simulink model "gm_DUALportRAMinterface_v3"  (R2024a)
settings: Solver=FixedStepDiscrete  StartTime=0.0  StopTime=20  RelTol=1e-3
undefined symbols (not defined in the file or in its folder): magnitude, Ts
libraries: hdlsllib x226, hdlmdlgenlib x102, embmathops x6, simulink x1, dsphdlxfrm2 x1
(part 5 of 6)

== system gm_DUALportRAMinterface_v3/PL/integration_block1/accumulator_scorer/64bitmsb_finder/8bit_PE10 ==
  D7 : Inport  OutDataTypeStr=boolean  PortDimensions=1  SampleTime=3.00000003e-08
  D6 : Inport  Port=2  OutDataTypeStr=boolean  PortDimensions=1  SampleTime=3.00000003e-08
  D5 : Inport  Port=3  OutDataTypeStr=boolean  PortDimensions=1  SampleTime=3.00000003e-08
  D4 : Inport  Port=4  OutDataTypeStr=boolean  PortDimensions=1  SampleTime=3.00000003e-08
  D3 : Inport  Port=5  OutDataTypeStr=boolean  PortDimensions=1  SampleTime=3.00000003e-08
  D2 : Inport  Port=6  OutDataTypeStr=boolean  PortDimensions=1  SampleTime=3.00000003e-08
  D1 : Inport  Port=7  OutDataTypeStr=boolean  PortDimensions=1  SampleTime=3.00000003e-08
  D0 : Inport  Port=8  OutDataTypeStr=boolean  PortDimensions=1  SampleTime=3.00000003e-08
  Add : Sum  OutDataTypeStr=fixdt(0, 5, 0)
  Bit Concat : hdlsllib/Logic and Bit Operations/Bit Concat  numInputs=3
  Constant2 : Constant  OutDataTypeStr=fixdt(0,4,0)  SampleTime=Ts
  Constant3 : Constant  Value=0  OutDataTypeStr=fixdt(0,4,0)  SampleTime=Ts
  Logical Operator{,10..16,22} (9 alike) : Logic  Operator=NOT  IconShape=distinctive  AllPortsSameDT=off  OutDataTypeStr=boolean
  Logical Operator1 : Logic  Operator=NAND  IconShape=distinctive  AllPortsSameDT=off  OutDataTypeStr=boolean
  Logical Operator{17..20} (4 alike) : Logic  Operator=OR  Inputs=4  IconShape=distinctive  AllPortsSameDT=off  OutDataTypeStr=boolean
  Logical Operator2 : Logic  Operator=NAND  Inputs=4  IconShape=distinctive  AllPortsSameDT=off  OutDataTypeStr=boolean
  Logical Operator21 : Logic  Operator=NAND  Inputs=3  IconShape=distinctive  AllPortsSameDT=off  OutDataTypeStr=boolean
  Logical Operator23 : Logic  IconShape=distinctive  AllPortsSameDT=off  OutDataTypeStr=boolean
  Logical Operator3 : Logic  Operator=NAND  Inputs=3  IconShape=distinctive  AllPortsSameDT=off  OutDataTypeStr=boolean
  Logical Operator4 : Logic  Inputs=3  IconShape=distinctive  AllPortsSameDT=off  OutDataTypeStr=boolean
  Logical Operator5 : Logic  Inputs=3  IconShape=distinctive  AllPortsSameDT=off  OutDataTypeStr=boolean
  Logical Operator6 : Logic  Inputs=4  IconShape=distinctive  AllPortsSameDT=off  OutDataTypeStr=boolean
  Logical Operator7 : Logic  Operator=NAND  Inputs=3  IconShape=distinctive  AllPortsSameDT=off  OutDataTypeStr=boolean
  Logical Operator8 : Logic  Operator=NAND  Inputs=4  IconShape=distinctive  AllPortsSameDT=off  OutDataTypeStr=boolean
  Logical Operator9 : Logic  Operator=NAND  Inputs=4  IconShape=distinctive  AllPortsSameDT=off  OutDataTypeStr=boolean
  Switch : Switch  Criteria=u2 > Threshold  OutDataTypeStr=fixdt(0, 4, 0)  SaturateOnIntegerOverflow=off  InputSameDT=off
  data2 : Outport  SampleTime=3.00000003e-08
  valid : Outport  Port=2  SampleTime=3.00000003e-08
  wires:
  D7/1 -> Logical Operator/1
  D6/1 -> Logical Operator1/2
  D5/1 -> Logical Operator3/3
  D4/1 -> Logical Operator2/4
  D3/1 -> Logical Operator7/3
  D2/1 -> Logical Operator8/4
  D1/1 -> Logical Operator9/4
  D0/1 -> Logical Operator20/2
  Add/1 -> data2/1
  Bit Concat/1 -> Add/2
  Constant2/1 -> Switch/3
  Constant3/1 -> Switch/1
  Logical Operator/1 -> Logical Operator6/3, Logical Operator5/3, Logical Operator4/3, Logical Operator3/2, Logical Operator2/3, Logical Operator10/1, Logical Operator1/1
  Logical Operator1/1 -> Logical Operator6/2, Logical Operator5/2, Logical Operator4/2, Logical Operator3/1, Logical Operator2/2, Logical Operator11/1
  Logical Operator10/1 -> Logical Operator19/1, Logical Operator18/1, Logical Operator17/1
  Logical Operator11/1 -> Logical Operator18/2, Logical Operator17/2
  Logical Operator12/1 -> Logical Operator19/2, Logical Operator17/3
  Logical Operator13/1 -> Logical Operator17/4
  Logical Operator14/1 -> Logical Operator19/4, Logical Operator18/3
  Logical Operator15/1 -> Logical Operator18/4
  Logical Operator16/1 -> Logical Operator19/3
  Logical Operator17/1 -> Logical Operator21/1, Logical Operator20/1, Bit Concat/1
  Logical Operator18/1 -> Logical Operator21/2, Logical Operator20/3, Bit Concat/2
  Logical Operator19/1 -> Logical Operator21/3, Logical Operator20/4, Bit Concat/3
  Logical Operator2/1 -> Logical Operator8/2, Logical Operator7/2, Logical Operator6/4, Logical Operator13/1
  Logical Operator20/1 -> Logical Operator22/1, valid/1
  Logical Operator21/1 -> Logical Operator23/1
  Logical Operator22/1 -> Logical Operator23/2
  Logical Operator23/1 -> Switch/2
  Logical Operator3/1 -> Logical Operator6/1, Logical Operator5/1, Logical Operator4/1, Logical Operator2/1, Logical Operator12/1
  Logical Operator4/1 -> Logical Operator7/1
  Logical Operator5/1 -> Logical Operator8/1
  Logical Operator6/1 -> Logical Operator9/1
  Logical Operator7/1 -> Logical Operator9/2, Logical Operator8/3, Logical Operator14/1
  Logical Operator8/1 -> Logical Operator9/3, Logical Operator15/1
  Logical Operator9/1 -> Logical Operator16/1
  Switch/1 -> Add/1

== system gm_DUALportRAMinterface_v3/PL/integration_block1/accumulator_scorer/64bitmsb_finder/8bit_PE2 ==
  D7 : Inport  OutDataTypeStr=fixdt(0, 1, 0)  PortDimensions=1  SampleTime=3.00000003e-08
  D6 : Inport  Port=2  OutDataTypeStr=fixdt(0, 1, 0)  PortDimensions=1  SampleTime=3.00000003e-08
  D5 : Inport  Port=3  OutDataTypeStr=fixdt(0, 1, 0)  PortDimensions=1  SampleTime=3.00000003e-08
  D4 : Inport  Port=4  OutDataTypeStr=fixdt(0, 1, 0)  PortDimensions=1  SampleTime=3.00000003e-08
  D3 : Inport  Port=5  OutDataTypeStr=fixdt(0, 1, 0)  PortDimensions=1  SampleTime=3.00000003e-08
  D2 : Inport  Port=6  OutDataTypeStr=fixdt(0, 1, 0)  PortDimensions=1  SampleTime=3.00000003e-08
  D1 : Inport  Port=7  OutDataTypeStr=fixdt(0, 1, 0)  PortDimensions=1  SampleTime=3.00000003e-08
  D0 : Inport  Port=8  OutDataTypeStr=fixdt(0, 1, 0)  PortDimensions=1  SampleTime=3.00000003e-08
  Add : Sum  OutDataTypeStr=fixdt(0, 5, 0)
  Bit Concat : hdlsllib/Logic and Bit Operations/Bit Concat  numInputs=3
  Constant2 : Constant  OutDataTypeStr=fixdt(0,4,0)  SampleTime=Ts
  Constant3 : Constant  Value=0  OutDataTypeStr=fixdt(0,4,0)  SampleTime=Ts
  Logical Operator{,10..16,22} (9 alike) : Logic  Operator=NOT  IconShape=distinctive  AllPortsSameDT=off  OutDataTypeStr=boolean
  Logical Operator1 : Logic  Operator=NAND  IconShape=distinctive  AllPortsSameDT=off  OutDataTypeStr=boolean
  Logical Operator{17..20} (4 alike) : Logic  Operator=OR  Inputs=4  IconShape=distinctive  AllPortsSameDT=off  OutDataTypeStr=boolean
  Logical Operator2 : Logic  Operator=NAND  Inputs=4  IconShape=distinctive  AllPortsSameDT=off  OutDataTypeStr=boolean
  Logical Operator21 : Logic  Operator=NAND  Inputs=3  IconShape=distinctive  AllPortsSameDT=off  OutDataTypeStr=boolean
  Logical Operator23 : Logic  IconShape=distinctive  AllPortsSameDT=off  OutDataTypeStr=boolean
  Logical Operator3 : Logic  Operator=NAND  Inputs=3  IconShape=distinctive  AllPortsSameDT=off  OutDataTypeStr=boolean
  Logical Operator4 : Logic  Inputs=3  IconShape=distinctive  AllPortsSameDT=off  OutDataTypeStr=boolean
  Logical Operator5 : Logic  Inputs=3  IconShape=distinctive  AllPortsSameDT=off  OutDataTypeStr=boolean
  Logical Operator6 : Logic  Inputs=4  IconShape=distinctive  AllPortsSameDT=off  OutDataTypeStr=boolean
  Logical Operator7 : Logic  Operator=NAND  Inputs=3  IconShape=distinctive  AllPortsSameDT=off  OutDataTypeStr=boolean
  Logical Operator8 : Logic  Operator=NAND  Inputs=4  IconShape=distinctive  AllPortsSameDT=off  OutDataTypeStr=boolean
  Logical Operator9 : Logic  Operator=NAND  Inputs=4  IconShape=distinctive  AllPortsSameDT=off  OutDataTypeStr=boolean
  Switch : Switch  Criteria=u2 > Threshold  OutDataTypeStr=fixdt(0, 4, 0)  SaturateOnIntegerOverflow=off  InputSameDT=off
  data2 : Outport  SampleTime=3.00000003e-08
  valid : Outport  Port=2  SampleTime=3.00000003e-08
  wires:
  D7/1 -> Logical Operator/1
  D6/1 -> Logical Operator1/2
  D5/1 -> Logical Operator3/3
  D4/1 -> Logical Operator2/4
  D3/1 -> Logical Operator7/3
  D2/1 -> Logical Operator8/4
  D1/1 -> Logical Operator9/4
  D0/1 -> Logical Operator20/2
  Add/1 -> data2/1
  Bit Concat/1 -> Add/2
  Constant2/1 -> Switch/3
  Constant3/1 -> Switch/1
  Logical Operator/1 -> Logical Operator6/3, Logical Operator5/3, Logical Operator4/3, Logical Operator3/2, Logical Operator2/3, Logical Operator10/1, Logical Operator1/1
  Logical Operator1/1 -> Logical Operator6/2, Logical Operator5/2, Logical Operator4/2, Logical Operator3/1, Logical Operator2/2, Logical Operator11/1
  Logical Operator10/1 -> Logical Operator19/1, Logical Operator18/1, Logical Operator17/1
  Logical Operator11/1 -> Logical Operator18/2, Logical Operator17/2
  Logical Operator12/1 -> Logical Operator19/2, Logical Operator17/3
  Logical Operator13/1 -> Logical Operator17/4
  Logical Operator14/1 -> Logical Operator19/4, Logical Operator18/3
  Logical Operator15/1 -> Logical Operator18/4
  Logical Operator16/1 -> Logical Operator19/3
  Logical Operator17/1 -> Logical Operator21/1, Logical Operator20/1, Bit Concat/1
  Logical Operator18/1 -> Logical Operator21/2, Logical Operator20/3, Bit Concat/2
  Logical Operator19/1 -> Logical Operator21/3, Logical Operator20/4, Bit Concat/3
  Logical Operator2/1 -> Logical Operator8/2, Logical Operator7/2, Logical Operator6/4, Logical Operator13/1
  Logical Operator20/1 -> Logical Operator22/1, valid/1
  Logical Operator21/1 -> Logical Operator23/1
  Logical Operator22/1 -> Logical Operator23/2
  Logical Operator23/1 -> Switch/2
  Logical Operator3/1 -> Logical Operator6/1, Logical Operator5/1, Logical Operator4/1, Logical Operator2/1, Logical Operator12/1
  Logical Operator4/1 -> Logical Operator7/1
  Logical Operator5/1 -> Logical Operator8/1
  Logical Operator6/1 -> Logical Operator9/1
  Logical Operator7/1 -> Logical Operator9/2, Logical Operator8/3, Logical Operator14/1
  Logical Operator8/1 -> Logical Operator9/3, Logical Operator15/1
  Logical Operator9/1 -> Logical Operator16/1
  Switch/1 -> Add/1

== system gm_DUALportRAMinterface_v3/PL/integration_block1/accumulator_scorer/64bitmsb_finder/8bit_PE3 ==
  D7 : Inport  OutDataTypeStr=fixdt(0, 1, 0)  PortDimensions=1  SampleTime=3.00000003e-08
  D6 : Inport  Port=2  OutDataTypeStr=fixdt(0, 1, 0)  PortDimensions=1  SampleTime=3.00000003e-08
  D5 : Inport  Port=3  OutDataTypeStr=fixdt(0, 1, 0)  PortDimensions=1  SampleTime=3.00000003e-08
  D4 : Inport  Port=4  OutDataTypeStr=fixdt(0, 1, 0)  PortDimensions=1  SampleTime=3.00000003e-08
  D3 : Inport  Port=5  OutDataTypeStr=fixdt(0, 1, 0)  PortDimensions=1  SampleTime=3.00000003e-08
  D2 : Inport  Port=6  OutDataTypeStr=fixdt(0, 1, 0)  PortDimensions=1  SampleTime=3.00000003e-08
  D1 : Inport  Port=7  OutDataTypeStr=fixdt(0, 1, 0)  PortDimensions=1  SampleTime=3.00000003e-08
  D0 : Inport  Port=8  OutDataTypeStr=fixdt(0, 1, 0)  PortDimensions=1  SampleTime=3.00000003e-08
  Add : Sum  OutDataTypeStr=fixdt(0, 5, 0)
  Bit Concat : hdlsllib/Logic and Bit Operations/Bit Concat  numInputs=3
  Constant2 : Constant  OutDataTypeStr=fixdt(0,4,0)  SampleTime=Ts
  Constant3 : Constant  Value=0  OutDataTypeStr=fixdt(0,4,0)  SampleTime=Ts
  Logical Operator{,10..16,22} (9 alike) : Logic  Operator=NOT  IconShape=distinctive  AllPortsSameDT=off  OutDataTypeStr=boolean
  Logical Operator1 : Logic  Operator=NAND  IconShape=distinctive  AllPortsSameDT=off  OutDataTypeStr=boolean
  Logical Operator{17..20} (4 alike) : Logic  Operator=OR  Inputs=4  IconShape=distinctive  AllPortsSameDT=off  OutDataTypeStr=boolean
  Logical Operator2 : Logic  Operator=NAND  Inputs=4  IconShape=distinctive  AllPortsSameDT=off  OutDataTypeStr=boolean
  Logical Operator21 : Logic  Operator=NAND  Inputs=3  IconShape=distinctive  AllPortsSameDT=off  OutDataTypeStr=boolean
  Logical Operator23 : Logic  IconShape=distinctive  AllPortsSameDT=off  OutDataTypeStr=boolean
  Logical Operator3 : Logic  Operator=NAND  Inputs=3  IconShape=distinctive  AllPortsSameDT=off  OutDataTypeStr=boolean
  Logical Operator4 : Logic  Inputs=3  IconShape=distinctive  AllPortsSameDT=off  OutDataTypeStr=boolean
  Logical Operator5 : Logic  Inputs=3  IconShape=distinctive  AllPortsSameDT=off  OutDataTypeStr=boolean
  Logical Operator6 : Logic  Inputs=4  IconShape=distinctive  AllPortsSameDT=off  OutDataTypeStr=boolean
  Logical Operator7 : Logic  Operator=NAND  Inputs=3  IconShape=distinctive  AllPortsSameDT=off  OutDataTypeStr=boolean
  Logical Operator8 : Logic  Operator=NAND  Inputs=4  IconShape=distinctive  AllPortsSameDT=off  OutDataTypeStr=boolean
  Logical Operator9 : Logic  Operator=NAND  Inputs=4  IconShape=distinctive  AllPortsSameDT=off  OutDataTypeStr=boolean
  Switch : Switch  Criteria=u2 > Threshold  OutDataTypeStr=fixdt(0, 4, 0)  SaturateOnIntegerOverflow=off  InputSameDT=off
  data2 : Outport  SampleTime=3.00000003e-08
  valid : Outport  Port=2  SampleTime=3.00000003e-08
  wires:
  D7/1 -> Logical Operator/1
  D6/1 -> Logical Operator1/2
  D5/1 -> Logical Operator3/3
  D4/1 -> Logical Operator2/4
  D3/1 -> Logical Operator7/3
  D2/1 -> Logical Operator8/4
  D1/1 -> Logical Operator9/4
  D0/1 -> Logical Operator20/2
  Add/1 -> data2/1
  Bit Concat/1 -> Add/2
  Constant2/1 -> Switch/3
  Constant3/1 -> Switch/1
  Logical Operator/1 -> Logical Operator6/3, Logical Operator5/3, Logical Operator4/3, Logical Operator3/2, Logical Operator2/3, Logical Operator10/1, Logical Operator1/1
  Logical Operator1/1 -> Logical Operator6/2, Logical Operator5/2, Logical Operator4/2, Logical Operator3/1, Logical Operator2/2, Logical Operator11/1
  Logical Operator10/1 -> Logical Operator19/1, Logical Operator18/1, Logical Operator17/1
  Logical Operator11/1 -> Logical Operator18/2, Logical Operator17/2
  Logical Operator12/1 -> Logical Operator19/2, Logical Operator17/3
  Logical Operator13/1 -> Logical Operator17/4
  Logical Operator14/1 -> Logical Operator19/4, Logical Operator18/3
  Logical Operator15/1 -> Logical Operator18/4
  Logical Operator16/1 -> Logical Operator19/3
  Logical Operator17/1 -> Logical Operator21/1, Logical Operator20/1, Bit Concat/1
  Logical Operator18/1 -> Logical Operator21/2, Logical Operator20/3, Bit Concat/2
  Logical Operator19/1 -> Logical Operator21/3, Logical Operator20/4, Bit Concat/3
  Logical Operator2/1 -> Logical Operator8/2, Logical Operator7/2, Logical Operator6/4, Logical Operator13/1
  Logical Operator20/1 -> Logical Operator22/1, valid/1
  Logical Operator21/1 -> Logical Operator23/1
  Logical Operator22/1 -> Logical Operator23/2
  Logical Operator23/1 -> Switch/2
  Logical Operator3/1 -> Logical Operator6/1, Logical Operator5/1, Logical Operator4/1, Logical Operator2/1, Logical Operator12/1
  Logical Operator4/1 -> Logical Operator7/1
  Logical Operator5/1 -> Logical Operator8/1
  Logical Operator6/1 -> Logical Operator9/1
  Logical Operator7/1 -> Logical Operator9/2, Logical Operator8/3, Logical Operator14/1
  Logical Operator8/1 -> Logical Operator9/3, Logical Operator15/1
  Logical Operator9/1 -> Logical Operator16/1
  Switch/1 -> Add/1

== system gm_DUALportRAMinterface_v3/PL/integration_block1/accumulator_scorer/64bitmsb_finder/8bit_PE4 ==
  D7 : Inport  OutDataTypeStr=fixdt(0, 1, 0)  PortDimensions=1  SampleTime=3.00000003e-08
  D6 : Inport  Port=2  OutDataTypeStr=fixdt(0, 1, 0)  PortDimensions=1  SampleTime=3.00000003e-08
  D5 : Inport  Port=3  OutDataTypeStr=fixdt(0, 1, 0)  PortDimensions=1  SampleTime=3.00000003e-08
  D4 : Inport  Port=4  OutDataTypeStr=fixdt(0, 1, 0)  PortDimensions=1  SampleTime=3.00000003e-08
  D3 : Inport  Port=5  OutDataTypeStr=fixdt(0, 1, 0)  PortDimensions=1  SampleTime=3.00000003e-08
  D2 : Inport  Port=6  OutDataTypeStr=fixdt(0, 1, 0)  PortDimensions=1  SampleTime=3.00000003e-08
  D1 : Inport  Port=7  OutDataTypeStr=fixdt(0, 1, 0)  PortDimensions=1  SampleTime=3.00000003e-08
  D0 : Inport  Port=8  OutDataTypeStr=fixdt(0, 1, 0)  PortDimensions=1  SampleTime=3.00000003e-08
  Add : Sum  OutDataTypeStr=fixdt(0, 5, 0)
  Bit Concat : hdlsllib/Logic and Bit Operations/Bit Concat  numInputs=3
  Constant2 : Constant  OutDataTypeStr=fixdt(0,4,0)  SampleTime=Ts
  Constant3 : Constant  Value=0  OutDataTypeStr=fixdt(0,4,0)  SampleTime=Ts
  Logical Operator{,10..16,22} (9 alike) : Logic  Operator=NOT  IconShape=distinctive  AllPortsSameDT=off  OutDataTypeStr=boolean
  Logical Operator1 : Logic  Operator=NAND  IconShape=distinctive  AllPortsSameDT=off  OutDataTypeStr=boolean
  Logical Operator{17..20} (4 alike) : Logic  Operator=OR  Inputs=4  IconShape=distinctive  AllPortsSameDT=off  OutDataTypeStr=boolean
  Logical Operator2 : Logic  Operator=NAND  Inputs=4  IconShape=distinctive  AllPortsSameDT=off  OutDataTypeStr=boolean
  Logical Operator21 : Logic  Operator=NAND  Inputs=3  IconShape=distinctive  AllPortsSameDT=off  OutDataTypeStr=boolean
  Logical Operator23 : Logic  IconShape=distinctive  AllPortsSameDT=off  OutDataTypeStr=boolean
  Logical Operator3 : Logic  Operator=NAND  Inputs=3  IconShape=distinctive  AllPortsSameDT=off  OutDataTypeStr=boolean
  Logical Operator4 : Logic  Inputs=3  IconShape=distinctive  AllPortsSameDT=off  OutDataTypeStr=boolean
  Logical Operator5 : Logic  Inputs=3  IconShape=distinctive  AllPortsSameDT=off  OutDataTypeStr=boolean
  Logical Operator6 : Logic  Inputs=4  IconShape=distinctive  AllPortsSameDT=off  OutDataTypeStr=boolean
  Logical Operator7 : Logic  Operator=NAND  Inputs=3  IconShape=distinctive  AllPortsSameDT=off  OutDataTypeStr=boolean
  Logical Operator8 : Logic  Operator=NAND  Inputs=4  IconShape=distinctive  AllPortsSameDT=off  OutDataTypeStr=boolean
  Logical Operator9 : Logic  Operator=NAND  Inputs=4  IconShape=distinctive  AllPortsSameDT=off  OutDataTypeStr=boolean
  Switch : Switch  Criteria=u2 > Threshold  OutDataTypeStr=fixdt(0, 4, 0)  SaturateOnIntegerOverflow=off  InputSameDT=off
  data2 : Outport  SampleTime=3.00000003e-08
  valid : Outport  Port=2  SampleTime=3.00000003e-08
  wires:
  D7/1 -> Logical Operator/1
  D6/1 -> Logical Operator1/2
  D5/1 -> Logical Operator3/3
  D4/1 -> Logical Operator2/4
  D3/1 -> Logical Operator7/3
  D2/1 -> Logical Operator8/4
  D1/1 -> Logical Operator9/4
  D0/1 -> Logical Operator20/2
  Add/1 -> data2/1
  Bit Concat/1 -> Add/2
  Constant2/1 -> Switch/3
  Constant3/1 -> Switch/1
  Logical Operator/1 -> Logical Operator6/3, Logical Operator5/3, Logical Operator4/3, Logical Operator3/2, Logical Operator2/3, Logical Operator10/1, Logical Operator1/1
  Logical Operator1/1 -> Logical Operator6/2, Logical Operator5/2, Logical Operator4/2, Logical Operator3/1, Logical Operator2/2, Logical Operator11/1
  Logical Operator10/1 -> Logical Operator19/1, Logical Operator18/1, Logical Operator17/1
  Logical Operator11/1 -> Logical Operator18/2, Logical Operator17/2
  Logical Operator12/1 -> Logical Operator19/2, Logical Operator17/3
  Logical Operator13/1 -> Logical Operator17/4
  Logical Operator14/1 -> Logical Operator19/4, Logical Operator18/3
  Logical Operator15/1 -> Logical Operator18/4
  Logical Operator16/1 -> Logical Operator19/3
  Logical Operator17/1 -> Logical Operator21/1, Logical Operator20/1, Bit Concat/1
  Logical Operator18/1 -> Logical Operator21/2, Logical Operator20/3, Bit Concat/2
  Logical Operator19/1 -> Logical Operator21/3, Logical Operator20/4, Bit Concat/3
  Logical Operator2/1 -> Logical Operator8/2, Logical Operator7/2, Logical Operator6/4, Logical Operator13/1
  Logical Operator20/1 -> Logical Operator22/1, valid/1
  Logical Operator21/1 -> Logical Operator23/1
  Logical Operator22/1 -> Logical Operator23/2
  Logical Operator23/1 -> Switch/2
  Logical Operator3/1 -> Logical Operator6/1, Logical Operator5/1, Logical Operator4/1, Logical Operator2/1, Logical Operator12/1
  Logical Operator4/1 -> Logical Operator7/1
  Logical Operator5/1 -> Logical Operator8/1
  Logical Operator6/1 -> Logical Operator9/1
  Logical Operator7/1 -> Logical Operator9/2, Logical Operator8/3, Logical Operator14/1
  Logical Operator8/1 -> Logical Operator9/3, Logical Operator15/1
  Logical Operator9/1 -> Logical Operator16/1
  Switch/1 -> Add/1

== system gm_DUALportRAMinterface_v3/PL/integration_block1/accumulator_scorer/64bitmsb_finder/8bit_PE5 ==
  D7 : Inport  OutDataTypeStr=fixdt(0, 1, 0)  PortDimensions=1  SampleTime=3.00000003e-08
  D6 : Inport  Port=2  OutDataTypeStr=fixdt(0, 1, 0)  PortDimensions=1  SampleTime=3.00000003e-08
  D5 : Inport  Port=3  OutDataTypeStr=fixdt(0, 1, 0)  PortDimensions=1  SampleTime=3.00000003e-08
  D4 : Inport  Port=4  OutDataTypeStr=fixdt(0, 1, 0)  PortDimensions=1  SampleTime=3.00000003e-08
  D3 : Inport  Port=5  OutDataTypeStr=fixdt(0, 1, 0)  PortDimensions=1  SampleTime=3.00000003e-08
  D2 : Inport  Port=6  OutDataTypeStr=fixdt(0, 1, 0)  PortDimensions=1  SampleTime=3.00000003e-08
  D1 : Inport  Port=7  OutDataTypeStr=fixdt(0, 1, 0)  PortDimensions=1  SampleTime=3.00000003e-08
  D0 : Inport  Port=8  OutDataTypeStr=fixdt(0, 1, 0)  PortDimensions=1  SampleTime=3.00000003e-08
  Add : Sum  OutDataTypeStr=fixdt(0, 5, 0)
  Bit Concat : hdlsllib/Logic and Bit Operations/Bit Concat  numInputs=3
  Constant2 : Constant  OutDataTypeStr=fixdt(0,4,0)  SampleTime=Ts
  Constant3 : Constant  Value=0  OutDataTypeStr=fixdt(0,4,0)  SampleTime=Ts
  Logical Operator{,10..16,22} (9 alike) : Logic  Operator=NOT  IconShape=distinctive  AllPortsSameDT=off  OutDataTypeStr=boolean
  Logical Operator1 : Logic  Operator=NAND  IconShape=distinctive  AllPortsSameDT=off  OutDataTypeStr=boolean
  Logical Operator{17..20} (4 alike) : Logic  Operator=OR  Inputs=4  IconShape=distinctive  AllPortsSameDT=off  OutDataTypeStr=boolean
  Logical Operator2 : Logic  Operator=NAND  Inputs=4  IconShape=distinctive  AllPortsSameDT=off  OutDataTypeStr=boolean
  Logical Operator21 : Logic  Operator=NAND  Inputs=3  IconShape=distinctive  AllPortsSameDT=off  OutDataTypeStr=boolean
  Logical Operator23 : Logic  IconShape=distinctive  AllPortsSameDT=off  OutDataTypeStr=boolean
  Logical Operator3 : Logic  Operator=NAND  Inputs=3  IconShape=distinctive  AllPortsSameDT=off  OutDataTypeStr=boolean
  Logical Operator4 : Logic  Inputs=3  IconShape=distinctive  AllPortsSameDT=off  OutDataTypeStr=boolean
  Logical Operator5 : Logic  Inputs=3  IconShape=distinctive  AllPortsSameDT=off  OutDataTypeStr=boolean
  Logical Operator6 : Logic  Inputs=4  IconShape=distinctive  AllPortsSameDT=off  OutDataTypeStr=boolean
  Logical Operator7 : Logic  Operator=NAND  Inputs=3  IconShape=distinctive  AllPortsSameDT=off  OutDataTypeStr=boolean
  Logical Operator8 : Logic  Operator=NAND  Inputs=4  IconShape=distinctive  AllPortsSameDT=off  OutDataTypeStr=boolean
  Logical Operator9 : Logic  Operator=NAND  Inputs=4  IconShape=distinctive  AllPortsSameDT=off  OutDataTypeStr=boolean
  Switch : Switch  Criteria=u2 > Threshold  OutDataTypeStr=fixdt(0, 4, 0)  SaturateOnIntegerOverflow=off  InputSameDT=off
  data2 : Outport  SampleTime=3.00000003e-08
  valid : Outport  Port=2  SampleTime=3.00000003e-08
  wires:
  D7/1 -> Logical Operator/1
  D6/1 -> Logical Operator1/2
  D5/1 -> Logical Operator3/3
  D4/1 -> Logical Operator2/4
  D3/1 -> Logical Operator7/3
  D2/1 -> Logical Operator8/4
  D1/1 -> Logical Operator9/4
  D0/1 -> Logical Operator20/2
  Add/1 -> data2/1
  Bit Concat/1 -> Add/2
  Constant2/1 -> Switch/3
  Constant3/1 -> Switch/1
  Logical Operator/1 -> Logical Operator6/3, Logical Operator5/3, Logical Operator4/3, Logical Operator3/2, Logical Operator2/3, Logical Operator10/1, Logical Operator1/1
  Logical Operator1/1 -> Logical Operator6/2, Logical Operator5/2, Logical Operator4/2, Logical Operator3/1, Logical Operator2/2, Logical Operator11/1
  Logical Operator10/1 -> Logical Operator19/1, Logical Operator18/1, Logical Operator17/1
  Logical Operator11/1 -> Logical Operator18/2, Logical Operator17/2
  Logical Operator12/1 -> Logical Operator19/2, Logical Operator17/3
  Logical Operator13/1 -> Logical Operator17/4
  Logical Operator14/1 -> Logical Operator19/4, Logical Operator18/3
  Logical Operator15/1 -> Logical Operator18/4
  Logical Operator16/1 -> Logical Operator19/3
  Logical Operator17/1 -> Logical Operator21/1, Logical Operator20/1, Bit Concat/1
  Logical Operator18/1 -> Logical Operator21/2, Logical Operator20/3, Bit Concat/2
  Logical Operator19/1 -> Logical Operator21/3, Logical Operator20/4, Bit Concat/3
  Logical Operator2/1 -> Logical Operator8/2, Logical Operator7/2, Logical Operator6/4, Logical Operator13/1
  Logical Operator20/1 -> Logical Operator22/1, valid/1
  Logical Operator21/1 -> Logical Operator23/1
  Logical Operator22/1 -> Logical Operator23/2
  Logical Operator23/1 -> Switch/2
  Logical Operator3/1 -> Logical Operator6/1, Logical Operator5/1, Logical Operator4/1, Logical Operator2/1, Logical Operator12/1
  Logical Operator4/1 -> Logical Operator7/1
  Logical Operator5/1 -> Logical Operator8/1
  Logical Operator6/1 -> Logical Operator9/1
  Logical Operator7/1 -> Logical Operator9/2, Logical Operator8/3, Logical Operator14/1
  Logical Operator8/1 -> Logical Operator9/3, Logical Operator15/1
  Logical Operator9/1 -> Logical Operator16/1
  Switch/1 -> Add/1

== system gm_DUALportRAMinterface_v3/PL/integration_block1/accumulator_scorer/64bitmsb_finder/8bit_PE6 ==
  D7 : Inport  OutDataTypeStr=fixdt(0, 1, 0)  PortDimensions=1  SampleTime=3.00000003e-08
  D6 : Inport  Port=2  OutDataTypeStr=fixdt(0, 1, 0)  PortDimensions=1  SampleTime=3.00000003e-08
  D5 : Inport  Port=3  OutDataTypeStr=fixdt(0, 1, 0)  PortDimensions=1  SampleTime=3.00000003e-08
  D4 : Inport  Port=4  OutDataTypeStr=fixdt(0, 1, 0)  PortDimensions=1  SampleTime=3.00000003e-08
  D3 : Inport  Port=5  OutDataTypeStr=fixdt(0, 1, 0)  PortDimensions=1  SampleTime=3.00000003e-08
  D2 : Inport  Port=6  OutDataTypeStr=fixdt(0, 1, 0)  PortDimensions=1  SampleTime=3.00000003e-08
  D1 : Inport  Port=7  OutDataTypeStr=fixdt(0, 1, 0)  PortDimensions=1  SampleTime=3.00000003e-08
  D0 : Inport  Port=8  OutDataTypeStr=fixdt(0, 1, 0)  PortDimensions=1  SampleTime=3.00000003e-08
  Add : Sum  OutDataTypeStr=fixdt(0, 5, 0)
  Bit Concat : hdlsllib/Logic and Bit Operations/Bit Concat  numInputs=3
  Constant2 : Constant  OutDataTypeStr=fixdt(0,4,0)  SampleTime=Ts
  Constant3 : Constant  Value=0  OutDataTypeStr=fixdt(0,4,0)  SampleTime=Ts
  Logical Operator{,10..16,22} (9 alike) : Logic  Operator=NOT  IconShape=distinctive  AllPortsSameDT=off  OutDataTypeStr=boolean
  Logical Operator1 : Logic  Operator=NAND  IconShape=distinctive  AllPortsSameDT=off  OutDataTypeStr=boolean
  Logical Operator{17..20} (4 alike) : Logic  Operator=OR  Inputs=4  IconShape=distinctive  AllPortsSameDT=off  OutDataTypeStr=boolean
  Logical Operator2 : Logic  Operator=NAND  Inputs=4  IconShape=distinctive  AllPortsSameDT=off  OutDataTypeStr=boolean
  Logical Operator21 : Logic  Operator=NAND  Inputs=3  IconShape=distinctive  AllPortsSameDT=off  OutDataTypeStr=boolean
  Logical Operator23 : Logic  IconShape=distinctive  AllPortsSameDT=off  OutDataTypeStr=boolean
  Logical Operator3 : Logic  Operator=NAND  Inputs=3  IconShape=distinctive  AllPortsSameDT=off  OutDataTypeStr=boolean
  Logical Operator4 : Logic  Inputs=3  IconShape=distinctive  AllPortsSameDT=off  OutDataTypeStr=boolean
  Logical Operator5 : Logic  Inputs=3  IconShape=distinctive  AllPortsSameDT=off  OutDataTypeStr=boolean
  Logical Operator6 : Logic  Inputs=4  IconShape=distinctive  AllPortsSameDT=off  OutDataTypeStr=boolean
  Logical Operator7 : Logic  Operator=NAND  Inputs=3  IconShape=distinctive  AllPortsSameDT=off  OutDataTypeStr=boolean
  Logical Operator8 : Logic  Operator=NAND  Inputs=4  IconShape=distinctive  AllPortsSameDT=off  OutDataTypeStr=boolean
  Logical Operator9 : Logic  Operator=NAND  Inputs=4  IconShape=distinctive  AllPortsSameDT=off  OutDataTypeStr=boolean
  Switch : Switch  Criteria=u2 > Threshold  OutDataTypeStr=fixdt(0, 4, 0)  SaturateOnIntegerOverflow=off  InputSameDT=off
  data2 : Outport  SampleTime=3.00000003e-08
  valid : Outport  Port=2  SampleTime=3.00000003e-08
  wires:
  D7/1 -> Logical Operator/1
  D6/1 -> Logical Operator1/2
  D5/1 -> Logical Operator3/3
  D4/1 -> Logical Operator2/4
  D3/1 -> Logical Operator7/3
  D2/1 -> Logical Operator8/4
  D1/1 -> Logical Operator9/4
  D0/1 -> Logical Operator20/2
  Add/1 -> data2/1
  Bit Concat/1 -> Add/2
  Constant2/1 -> Switch/3
  Constant3/1 -> Switch/1
  Logical Operator/1 -> Logical Operator6/3, Logical Operator5/3, Logical Operator4/3, Logical Operator3/2, Logical Operator2/3, Logical Operator10/1, Logical Operator1/1
  Logical Operator1/1 -> Logical Operator6/2, Logical Operator5/2, Logical Operator4/2, Logical Operator3/1, Logical Operator2/2, Logical Operator11/1
  Logical Operator10/1 -> Logical Operator19/1, Logical Operator18/1, Logical Operator17/1
  Logical Operator11/1 -> Logical Operator18/2, Logical Operator17/2
  Logical Operator12/1 -> Logical Operator19/2, Logical Operator17/3
  Logical Operator13/1 -> Logical Operator17/4
  Logical Operator14/1 -> Logical Operator19/4, Logical Operator18/3
  Logical Operator15/1 -> Logical Operator18/4
  Logical Operator16/1 -> Logical Operator19/3
  Logical Operator17/1 -> Logical Operator21/1, Logical Operator20/1, Bit Concat/1
  Logical Operator18/1 -> Logical Operator21/2, Logical Operator20/3, Bit Concat/2
  Logical Operator19/1 -> Logical Operator21/3, Logical Operator20/4, Bit Concat/3
  Logical Operator2/1 -> Logical Operator8/2, Logical Operator7/2, Logical Operator6/4, Logical Operator13/1
  Logical Operator20/1 -> Logical Operator22/1, valid/1
  Logical Operator21/1 -> Logical Operator23/1
  Logical Operator22/1 -> Logical Operator23/2
  Logical Operator23/1 -> Switch/2
  Logical Operator3/1 -> Logical Operator6/1, Logical Operator5/1, Logical Operator4/1, Logical Operator2/1, Logical Operator12/1
  Logical Operator4/1 -> Logical Operator7/1
  Logical Operator5/1 -> Logical Operator8/1
  Logical Operator6/1 -> Logical Operator9/1
  Logical Operator7/1 -> Logical Operator9/2, Logical Operator8/3, Logical Operator14/1
  Logical Operator8/1 -> Logical Operator9/3, Logical Operator15/1
  Logical Operator9/1 -> Logical Operator16/1
  Switch/1 -> Add/1

== system gm_DUALportRAMinterface_v3/PL/integration_block1/accumulator_scorer/64bitmsb_finder/8bit_PE7 ==
  D7 : Inport  OutDataTypeStr=fixdt(0, 1, 0)  PortDimensions=1  SampleTime=3.00000003e-08
  D6 : Inport  Port=2  OutDataTypeStr=fixdt(0, 1, 0)  PortDimensions=1  SampleTime=3.00000003e-08
  D5 : Inport  Port=3  OutDataTypeStr=fixdt(0, 1, 0)  PortDimensions=1  SampleTime=3.00000003e-08
  D4 : Inport  Port=4  OutDataTypeStr=fixdt(0, 1, 0)  PortDimensions=1  SampleTime=3.00000003e-08
  D3 : Inport  Port=5  OutDataTypeStr=fixdt(0, 1, 0)  PortDimensions=1  SampleTime=3.00000003e-08
  D2 : Inport  Port=6  OutDataTypeStr=fixdt(0, 1, 0)  PortDimensions=1  SampleTime=3.00000003e-08
  D1 : Inport  Port=7  OutDataTypeStr=fixdt(0, 1, 0)  PortDimensions=1  SampleTime=3.00000003e-08
  D0 : Inport  Port=8  OutDataTypeStr=fixdt(0, 1, 0)  PortDimensions=1  SampleTime=3.00000003e-08
  Add : Sum  OutDataTypeStr=fixdt(0, 5, 0)
  Bit Concat : hdlsllib/Logic and Bit Operations/Bit Concat  numInputs=3
  Constant2 : Constant  OutDataTypeStr=fixdt(0,4,0)  SampleTime=Ts
  Constant3 : Constant  Value=0  OutDataTypeStr=fixdt(0,4,0)  SampleTime=Ts
  Logical Operator{,10..16,22} (9 alike) : Logic  Operator=NOT  IconShape=distinctive  AllPortsSameDT=off  OutDataTypeStr=boolean
  Logical Operator1 : Logic  Operator=NAND  IconShape=distinctive  AllPortsSameDT=off  OutDataTypeStr=boolean
  Logical Operator{17..20} (4 alike) : Logic  Operator=OR  Inputs=4  IconShape=distinctive  AllPortsSameDT=off  OutDataTypeStr=boolean
  Logical Operator2 : Logic  Operator=NAND  Inputs=4  IconShape=distinctive  AllPortsSameDT=off  OutDataTypeStr=boolean
  Logical Operator21 : Logic  Operator=NAND  Inputs=3  IconShape=distinctive  AllPortsSameDT=off  OutDataTypeStr=boolean
  Logical Operator23 : Logic  IconShape=distinctive  AllPortsSameDT=off  OutDataTypeStr=boolean
  Logical Operator3 : Logic  Operator=NAND  Inputs=3  IconShape=distinctive  AllPortsSameDT=off  OutDataTypeStr=boolean
  Logical Operator4 : Logic  Inputs=3  IconShape=distinctive  AllPortsSameDT=off  OutDataTypeStr=boolean
  Logical Operator5 : Logic  Inputs=3  IconShape=distinctive  AllPortsSameDT=off  OutDataTypeStr=boolean
  Logical Operator6 : Logic  Inputs=4  IconShape=distinctive  AllPortsSameDT=off  OutDataTypeStr=boolean
  Logical Operator7 : Logic  Operator=NAND  Inputs=3  IconShape=distinctive  AllPortsSameDT=off  OutDataTypeStr=boolean
  Logical Operator8 : Logic  Operator=NAND  Inputs=4  IconShape=distinctive  AllPortsSameDT=off  OutDataTypeStr=boolean
  Logical Operator9 : Logic  Operator=NAND  Inputs=4  IconShape=distinctive  AllPortsSameDT=off  OutDataTypeStr=boolean
  Switch : Switch  Criteria=u2 > Threshold  OutDataTypeStr=fixdt(0, 4, 0)  SaturateOnIntegerOverflow=off  InputSameDT=off
  data2 : Outport  SampleTime=3.00000003e-08
  valid : Outport  Port=2  SampleTime=3.00000003e-08
  wires:
  D7/1 -> Logical Operator/1
  D6/1 -> Logical Operator1/2
  D5/1 -> Logical Operator3/3
  D4/1 -> Logical Operator2/4
  D3/1 -> Logical Operator7/3
  D2/1 -> Logical Operator8/4
  D1/1 -> Logical Operator9/4
  D0/1 -> Logical Operator20/2
  Add/1 -> data2/1
  Bit Concat/1 -> Add/2
  Constant2/1 -> Switch/3
  Constant3/1 -> Switch/1
  Logical Operator/1 -> Logical Operator6/3, Logical Operator5/3, Logical Operator4/3, Logical Operator3/2, Logical Operator2/3, Logical Operator10/1, Logical Operator1/1
  Logical Operator1/1 -> Logical Operator6/2, Logical Operator5/2, Logical Operator4/2, Logical Operator3/1, Logical Operator2/2, Logical Operator11/1
  Logical Operator10/1 -> Logical Operator19/1, Logical Operator18/1, Logical Operator17/1
  Logical Operator11/1 -> Logical Operator18/2, Logical Operator17/2
  Logical Operator12/1 -> Logical Operator19/2, Logical Operator17/3
  Logical Operator13/1 -> Logical Operator17/4
  Logical Operator14/1 -> Logical Operator19/4, Logical Operator18/3
  Logical Operator15/1 -> Logical Operator18/4
  Logical Operator16/1 -> Logical Operator19/3
  Logical Operator17/1 -> Logical Operator21/1, Logical Operator20/1, Bit Concat/1
  Logical Operator18/1 -> Logical Operator21/2, Logical Operator20/3, Bit Concat/2
  Logical Operator19/1 -> Logical Operator21/3, Logical Operator20/4, Bit Concat/3
  Logical Operator2/1 -> Logical Operator8/2, Logical Operator7/2, Logical Operator6/4, Logical Operator13/1
  Logical Operator20/1 -> Logical Operator22/1, valid/1
  Logical Operator21/1 -> Logical Operator23/1
  Logical Operator22/1 -> Logical Operator23/2
  Logical Operator23/1 -> Switch/2
  Logical Operator3/1 -> Logical Operator6/1, Logical Operator5/1, Logical Operator4/1, Logical Operator2/1, Logical Operator12/1
  Logical Operator4/1 -> Logical Operator7/1
  Logical Operator5/1 -> Logical Operator8/1
  Logical Operator6/1 -> Logical Operator9/1
  Logical Operator7/1 -> Logical Operator9/2, Logical Operator8/3, Logical Operator14/1
  Logical Operator8/1 -> Logical Operator9/3, Logical Operator15/1
  Logical Operator9/1 -> Logical Operator16/1
  Switch/1 -> Add/1

== system gm_DUALportRAMinterface_v3/PL/integration_block1/accumulator_scorer/64bitmsb_finder/8bit_PE8 ==
  D7 : Inport  OutDataTypeStr=fixdt(0, 1, 0)  PortDimensions=1  SampleTime=3.00000003e-08
  D6 : Inport  Port=2  OutDataTypeStr=fixdt(0, 1, 0)  PortDimensions=1  SampleTime=3.00000003e-08
  D5 : Inport  Port=3  OutDataTypeStr=fixdt(0, 1, 0)  PortDimensions=1  SampleTime=3.00000003e-08
  D4 : Inport  Port=4  OutDataTypeStr=fixdt(0, 1, 0)  PortDimensions=1  SampleTime=3.00000003e-08
  D3 : Inport  Port=5  OutDataTypeStr=fixdt(0, 1, 0)  PortDimensions=1  SampleTime=3.00000003e-08
  D2 : Inport  Port=6  OutDataTypeStr=fixdt(0, 1, 0)  PortDimensions=1  SampleTime=3.00000003e-08
  D1 : Inport  Port=7  OutDataTypeStr=fixdt(0, 1, 0)  PortDimensions=1  SampleTime=3.00000003e-08
  D0 : Inport  Port=8  OutDataTypeStr=fixdt(0, 1, 0)  PortDimensions=1  SampleTime=3.00000003e-08
  Add : Sum  OutDataTypeStr=fixdt(0, 5, 0)
  Bit Concat : hdlsllib/Logic and Bit Operations/Bit Concat  numInputs=3
  Constant2 : Constant  OutDataTypeStr=fixdt(0,4,0)  SampleTime=Ts
  Constant3 : Constant  Value=0  OutDataTypeStr=fixdt(0,4,0)  SampleTime=Ts
  Logical Operator{,10..16,22} (9 alike) : Logic  Operator=NOT  IconShape=distinctive  AllPortsSameDT=off  OutDataTypeStr=boolean
  Logical Operator1 : Logic  Operator=NAND  IconShape=distinctive  AllPortsSameDT=off  OutDataTypeStr=boolean
  Logical Operator{17..20} (4 alike) : Logic  Operator=OR  Inputs=4  IconShape=distinctive  AllPortsSameDT=off  OutDataTypeStr=boolean
  Logical Operator2 : Logic  Operator=NAND  Inputs=4  IconShape=distinctive  AllPortsSameDT=off  OutDataTypeStr=boolean
  Logical Operator21 : Logic  Operator=NAND  Inputs=3  IconShape=distinctive  AllPortsSameDT=off  OutDataTypeStr=boolean
  Logical Operator23 : Logic  IconShape=distinctive  AllPortsSameDT=off  OutDataTypeStr=boolean
  Logical Operator3 : Logic  Operator=NAND  Inputs=3  IconShape=distinctive  AllPortsSameDT=off  OutDataTypeStr=boolean
  Logical Operator4 : Logic  Inputs=3  IconShape=distinctive  AllPortsSameDT=off  OutDataTypeStr=boolean
  Logical Operator5 : Logic  Inputs=3  IconShape=distinctive  AllPortsSameDT=off  OutDataTypeStr=boolean
  Logical Operator6 : Logic  Inputs=4  IconShape=distinctive  AllPortsSameDT=off  OutDataTypeStr=boolean
  Logical Operator7 : Logic  Operator=NAND  Inputs=3  IconShape=distinctive  AllPortsSameDT=off  OutDataTypeStr=boolean
  Logical Operator8 : Logic  Operator=NAND  Inputs=4  IconShape=distinctive  AllPortsSameDT=off  OutDataTypeStr=boolean
  Logical Operator9 : Logic  Operator=NAND  Inputs=4  IconShape=distinctive  AllPortsSameDT=off  OutDataTypeStr=boolean
  Switch : Switch  Criteria=u2 > Threshold  OutDataTypeStr=fixdt(0, 4, 0)  SaturateOnIntegerOverflow=off  InputSameDT=off
  data2 : Outport  SampleTime=3.00000003e-08
  valid : Outport  Port=2  SampleTime=3.00000003e-08
  wires:
  D7/1 -> Logical Operator/1
  D6/1 -> Logical Operator1/2
  D5/1 -> Logical Operator3/3
  D4/1 -> Logical Operator2/4
  D3/1 -> Logical Operator7/3
  D2/1 -> Logical Operator8/4
  D1/1 -> Logical Operator9/4
  D0/1 -> Logical Operator20/2
  Add/1 -> data2/1
  Bit Concat/1 -> Add/2
  Constant2/1 -> Switch/3
  Constant3/1 -> Switch/1
  Logical Operator/1 -> Logical Operator6/3, Logical Operator5/3, Logical Operator4/3, Logical Operator3/2, Logical Operator2/3, Logical Operator10/1, Logical Operator1/1
  Logical Operator1/1 -> Logical Operator6/2, Logical Operator5/2, Logical Operator4/2, Logical Operator3/1, Logical Operator2/2, Logical Operator11/1
  Logical Operator10/1 -> Logical Operator19/1, Logical Operator18/1, Logical Operator17/1
  Logical Operator11/1 -> Logical Operator18/2, Logical Operator17/2
  Logical Operator12/1 -> Logical Operator19/2, Logical Operator17/3
  Logical Operator13/1 -> Logical Operator17/4
  Logical Operator14/1 -> Logical Operator19/4, Logical Operator18/3
  Logical Operator15/1 -> Logical Operator18/4
  Logical Operator16/1 -> Logical Operator19/3
  Logical Operator17/1 -> Logical Operator21/1, Logical Operator20/1, Bit Concat/1
  Logical Operator18/1 -> Logical Operator21/2, Logical Operator20/3, Bit Concat/2
  Logical Operator19/1 -> Logical Operator21/3, Logical Operator20/4, Bit Concat/3
  Logical Operator2/1 -> Logical Operator8/2, Logical Operator7/2, Logical Operator6/4, Logical Operator13/1
  Logical Operator20/1 -> Logical Operator22/1, valid/1
  Logical Operator21/1 -> Logical Operator23/1
  Logical Operator22/1 -> Logical Operator23/2
  Logical Operator23/1 -> Switch/2
  Logical Operator3/1 -> Logical Operator6/1, Logical Operator5/1, Logical Operator4/1, Logical Operator2/1, Logical Operator12/1
  Logical Operator4/1 -> Logical Operator7/1
  Logical Operator5/1 -> Logical Operator8/1
  Logical Operator6/1 -> Logical Operator9/1
  Logical Operator7/1 -> Logical Operator9/2, Logical Operator8/3, Logical Operator14/1
  Logical Operator8/1 -> Logical Operator9/3, Logical Operator15/1
  Logical Operator9/1 -> Logical Operator16/1
  Switch/1 -> Add/1

== system gm_DUALportRAMinterface_v3/PL/integration_block1/GA_main/coefficent_array/individual1/Subsystem ==
  reg_in : Inport  OutDataTypeStr=fixdt(1, 33, 15)  PortDimensions=1  SampleTime=3.00000003e-08
  enable : Inport  Port=2  OutDataTypeStr=boolean  PortDimensions=1  SampleTime=3.00000003e-08
  Delay : Delay  DelayLength=1  InitialCondition=0  SampleTime=Ts
  Switch : Switch  Criteria=u2 > Threshold  OutDataTypeStr=fixdt(1, 33, 15)  SaturateOnIntegerOverflow=off  InputSameDT=off
  reg_out : Outport  SampleTime=3.00000003e-08
  wires:
  Delay/1 -> reg_out/1, Switch/3
  reg_in/1 -> Switch/1
  enable/1 -> Switch/2
  Switch/1 -> Delay/1

== system gm_DUALportRAMinterface_v3/PL/integration_block1/GA_main/coefficent_array/individual1/Subsystem1 ==
  reg_in : Inport  OutDataTypeStr=fixdt(1, 33, 15)  PortDimensions=1  SampleTime=3.00000003e-08
  enable : Inport  Port=2  OutDataTypeStr=boolean  PortDimensions=1  SampleTime=3.00000003e-08
  Delay : Delay  DelayLength=1  InitialCondition=0  SampleTime=Ts
  Switch : Switch  Criteria=u2 > Threshold  OutDataTypeStr=fixdt(1, 33, 15)  SaturateOnIntegerOverflow=off  InputSameDT=off
  reg_out : Outport  SampleTime=3.00000003e-08
  wires:
  Delay/1 -> reg_out/1, Switch/3
  reg_in/1 -> Switch/1
  enable/1 -> Switch/2
  Switch/1 -> Delay/1

== system gm_DUALportRAMinterface_v3/PL/integration_block1/GA_main/coefficent_array/individual1/Subsystem2 ==
  reg_in : Inport  OutDataTypeStr=fixdt(1, 33, 15)  PortDimensions=1  SampleTime=3.00000003e-08
  enable : Inport  Port=2  OutDataTypeStr=boolean  PortDimensions=1  SampleTime=3.00000003e-08
  Delay : Delay  DelayLength=1  InitialCondition=0  SampleTime=Ts
  Switch : Switch  Criteria=u2 > Threshold  OutDataTypeStr=fixdt(1, 33, 15)  SaturateOnIntegerOverflow=off  InputSameDT=off
  reg_out : Outport  SampleTime=3.00000003e-08
  wires:
  Delay/1 -> reg_out/1, Switch/3
  reg_in/1 -> Switch/1
  enable/1 -> Switch/2
  Switch/1 -> Delay/1

== system gm_DUALportRAMinterface_v3/PL/integration_block1/GA_main/coefficent_array/individual1/Subsystem3 ==
  reg_in : Inport  OutDataTypeStr=fixdt(1, 33, 15)  PortDimensions=1  SampleTime=3.00000003e-08
  enable : Inport  Port=2  OutDataTypeStr=boolean  PortDimensions=1  SampleTime=3.00000003e-08
  Delay : Delay  DelayLength=1  InitialCondition=0  SampleTime=Ts
  Switch : Switch  Criteria=u2 > Threshold  OutDataTypeStr=fixdt(1, 33, 15)  SaturateOnIntegerOverflow=off  InputSameDT=off
  reg_out : Outport  SampleTime=3.00000003e-08
  wires:
  Delay/1 -> reg_out/1, Switch/3
  reg_in/1 -> Switch/1
  enable/1 -> Switch/2
  Switch/1 -> Delay/1

== system gm_DUALportRAMinterface_v3/PL/integration_block1/GA_main/coefficent_array/individual1/Subsystem4 ==
  reg_in : Inport  OutDataTypeStr=fixdt(1, 33, 15)  PortDimensions=1  SampleTime=3.00000003e-08
  enable : Inport  Port=2  OutDataTypeStr=boolean  PortDimensions=1  SampleTime=3.00000003e-08
  Delay : Delay  DelayLength=1  InitialCondition=0  SampleTime=Ts
  Switch : Switch  Criteria=u2 > Threshold  OutDataTypeStr=fixdt(1, 33, 15)  SaturateOnIntegerOverflow=off  InputSameDT=off
  reg_out : Outport  SampleTime=3.00000003e-08
  wires:
  Delay/1 -> reg_out/1, Switch/3
  reg_in/1 -> Switch/1
  enable/1 -> Switch/2
  Switch/1 -> Delay/1

== system gm_DUALportRAMinterface_v3/PL/integration_block1/GA_main/coefficent_array/individual1/Subsystem5 ==
  reg_in : Inport  OutDataTypeStr=fixdt(1, 33, 15)  PortDimensions=1  SampleTime=3.00000003e-08
  enable : Inport  Port=2  OutDataTypeStr=boolean  PortDimensions=1  SampleTime=3.00000003e-08
  Delay : Delay  DelayLength=1  InitialCondition=0  SampleTime=Ts
  Switch : Switch  Criteria=u2 > Threshold  OutDataTypeStr=fixdt(1, 33, 15)  SaturateOnIntegerOverflow=off  InputSameDT=off
  reg_out : Outport  SampleTime=3.00000003e-08
  wires:
  Delay/1 -> reg_out/1, Switch/3
  reg_in/1 -> Switch/1
  enable/1 -> Switch/2
  Switch/1 -> Delay/1

== system gm_DUALportRAMinterface_v3/PL/integration_block1/GA_main/coefficent_array/individual1/Subsystem6 ==
  reg_in : Inport  OutDataTypeStr=fixdt(1, 33, 15)  PortDimensions=1  SampleTime=3.00000003e-08
  enable : Inport  Port=2  OutDataTypeStr=boolean  PortDimensions=1  SampleTime=3.00000003e-08
  Delay : Delay  DelayLength=1  InitialCondition=0  SampleTime=Ts
  Switch : Switch  Criteria=u2 > Threshold  OutDataTypeStr=fixdt(1, 33, 15)  SaturateOnIntegerOverflow=off  InputSameDT=off
  reg_out : Outport  SampleTime=3.00000003e-08
  wires:
  Delay/1 -> reg_out/1, Switch/3
  reg_in/1 -> Switch/1
  enable/1 -> Switch/2
  Switch/1 -> Delay/1

== system gm_DUALportRAMinterface_v3/PL/integration_block1/GA_main/coefficent_array/individual2/Subsystem ==
  reg_in : Inport  OutDataTypeStr=fixdt(1, 33, 15)  PortDimensions=1  SampleTime=3.00000003e-08
  enable : Inport  Port=2  OutDataTypeStr=boolean  PortDimensions=1  SampleTime=3.00000003e-08
  Delay : Delay  DelayLength=1  InitialCondition=0  SampleTime=Ts
  Switch : Switch  Criteria=u2 > Threshold  OutDataTypeStr=fixdt(1, 33, 15)  SaturateOnIntegerOverflow=off  InputSameDT=off
  reg_out : Outport  SampleTime=3.00000003e-08
  wires:
  Delay/1 -> reg_out/1, Switch/3
  reg_in/1 -> Switch/1
  enable/1 -> Switch/2
  Switch/1 -> Delay/1

== system gm_DUALportRAMinterface_v3/PL/integration_block1/GA_main/coefficent_array/individual2/Subsystem1 ==
  reg_in : Inport  OutDataTypeStr=fixdt(1, 33, 15)  PortDimensions=1  SampleTime=3.00000003e-08
  enable : Inport  Port=2  OutDataTypeStr=boolean  PortDimensions=1  SampleTime=3.00000003e-08
  Delay : Delay  DelayLength=1  InitialCondition=0  SampleTime=Ts
  Switch : Switch  Criteria=u2 > Threshold  OutDataTypeStr=fixdt(1, 33, 15)  SaturateOnIntegerOverflow=off  InputSameDT=off
  reg_out : Outport  SampleTime=3.00000003e-08
  wires:
  Delay/1 -> reg_out/1, Switch/3
  reg_in/1 -> Switch/1
  enable/1 -> Switch/2
  Switch/1 -> Delay/1

== system gm_DUALportRAMinterface_v3/PL/integration_block1/GA_main/coefficent_array/individual2/Subsystem2 ==
  reg_in : Inport  OutDataTypeStr=fixdt(1, 33, 15)  PortDimensions=1  SampleTime=3.00000003e-08
  enable : Inport  Port=2  OutDataTypeStr=boolean  PortDimensions=1  SampleTime=3.00000003e-08
  Delay : Delay  DelayLength=1  InitialCondition=0  SampleTime=Ts
  Switch : Switch  Criteria=u2 > Threshold  OutDataTypeStr=fixdt(1, 33, 15)  SaturateOnIntegerOverflow=off  InputSameDT=off
  reg_out : Outport  SampleTime=3.00000003e-08
  wires:
  Delay/1 -> reg_out/1, Switch/3
  reg_in/1 -> Switch/1
  enable/1 -> Switch/2
  Switch/1 -> Delay/1

== system gm_DUALportRAMinterface_v3/PL/integration_block1/GA_main/coefficent_array/individual2/Subsystem3 ==
  reg_in : Inport  OutDataTypeStr=fixdt(1, 33, 15)  PortDimensions=1  SampleTime=3.00000003e-08
  enable : Inport  Port=2  OutDataTypeStr=boolean  PortDimensions=1  SampleTime=3.00000003e-08
  Delay : Delay  DelayLength=1  InitialCondition=0  SampleTime=Ts
  Switch : Switch  Criteria=u2 > Threshold  OutDataTypeStr=fixdt(1, 33, 15)  SaturateOnIntegerOverflow=off  InputSameDT=off
  reg_out : Outport  SampleTime=3.00000003e-08
  wires:
  Delay/1 -> reg_out/1, Switch/3
  reg_in/1 -> Switch/1
  enable/1 -> Switch/2
  Switch/1 -> Delay/1

== system gm_DUALportRAMinterface_v3/PL/integration_block1/GA_main/coefficent_array/individual2/Subsystem4 ==
  reg_in : Inport  OutDataTypeStr=fixdt(1, 33, 15)  PortDimensions=1  SampleTime=3.00000003e-08
  enable : Inport  Port=2  OutDataTypeStr=boolean  PortDimensions=1  SampleTime=3.00000003e-08
  Delay : Delay  DelayLength=1  InitialCondition=0  SampleTime=Ts
  Switch : Switch  Criteria=u2 > Threshold  OutDataTypeStr=fixdt(1, 33, 15)  SaturateOnIntegerOverflow=off  InputSameDT=off
  reg_out : Outport  SampleTime=3.00000003e-08
  wires:
  Delay/1 -> reg_out/1, Switch/3
  reg_in/1 -> Switch/1
  enable/1 -> Switch/2
  Switch/1 -> Delay/1

== system gm_DUALportRAMinterface_v3/PL/integration_block1/GA_main/coefficent_array/individual2/Subsystem5 ==
  reg_in : Inport  OutDataTypeStr=fixdt(1, 33, 15)  PortDimensions=1  SampleTime=3.00000003e-08
  enable : Inport  Port=2  OutDataTypeStr=boolean  PortDimensions=1  SampleTime=3.00000003e-08
  Delay : Delay  DelayLength=1  InitialCondition=0  SampleTime=Ts
  Switch : Switch  Criteria=u2 > Threshold  OutDataTypeStr=fixdt(1, 33, 15)  SaturateOnIntegerOverflow=off  InputSameDT=off
  reg_out : Outport  SampleTime=3.00000003e-08
  wires:
  Delay/1 -> reg_out/1, Switch/3
  reg_in/1 -> Switch/1
  enable/1 -> Switch/2
  Switch/1 -> Delay/1

== system gm_DUALportRAMinterface_v3/PL/integration_block1/GA_main/coefficent_array/individual2/Subsystem6 ==
  reg_in : Inport  OutDataTypeStr=fixdt(1, 33, 15)  PortDimensions=1  SampleTime=3.00000003e-08
  enable : Inport  Port=2  OutDataTypeStr=boolean  PortDimensions=1  SampleTime=3.00000003e-08
  Delay : Delay  DelayLength=1  InitialCondition=0  SampleTime=Ts
  Switch : Switch  Criteria=u2 > Threshold  OutDataTypeStr=fixdt(1, 33, 15)  SaturateOnIntegerOverflow=off  InputSameDT=off
  reg_out : Outport  SampleTime=3.00000003e-08
  wires:
  Delay/1 -> reg_out/1, Switch/3
  reg_in/1 -> Switch/1
  enable/1 -> Switch/2
  Switch/1 -> Delay/1
